simulink model "levitat_model"  (R2024b)
settings: Solver=VariableStepAuto  StartTime=0.0  StopTime=Tsim  RelTol=1e-3
values from neighbouring files (symbols this model uses):
  g = 9.81    [gen_simdata_levit.m]    (also in levitat_data.mat)
  ibar = sqrt((m*g*(mean(z1(idx_start:idx_end))-z0).^2-k0)/Km)    [gen_simdata_levit.m]    (also in levitat_data.mat = 0.990880956794)
  K = place(A,B,pcl)    [gen_simdata_levit.m]
  k0 = 0    [gen_simdata_levit.m]    (also in levitat_data.mat; levitat_id_flcmo.m = x(2))
  Km = magnet_params(1)    [gen_simdata_levit.m]    (also in levitat_data.mat = 0.000210393151874)
  Kt = transducer_params(1)    [gen_simdata_levit.m]    (also in levitat_data.mat = 655.477466063)
  m = 24.197e-3    (= 0.024197)    [gen_simdata_levit.m]    (also in levitat_data.mat)
  Ts = 1e-2    (= 0.01)    [gen_simdata_levit.m]    (also in levitat_data.mat; run_ls.m = d.Ts)
  v0 = transducer_params(2)    [gen_simdata_levit.m]    (also in levitat_data.mat = -40.6780019306)
  zini = z_bar + 2*epsilon*rand - epsilon    [gen_simdata_levit.m]
settings Model: Creator=simon  LastModifiedBy=simon
settings DebuggingCC: UnconnectedInputMsg=warning  UnconnectedOutputMsg=warning  UnconnectedLineMsg=warning
settings ModelReferenceCC: EnableRefExpFcnMdlSchedulingChecks=on
settings RTWCC: GPUComputeCapability=3.5  DLArmComputeVersion=19.05

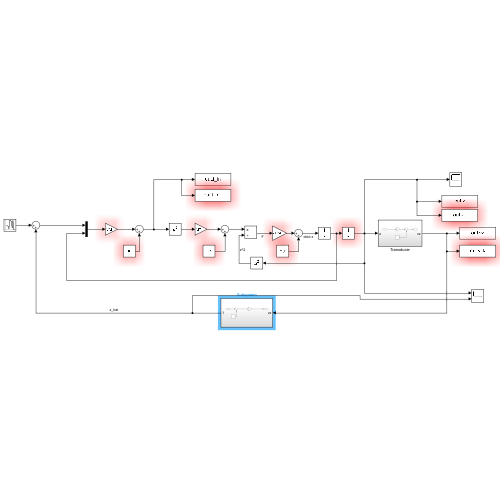
[thumbnail: Simulink's stored preview of the top-level diagram]
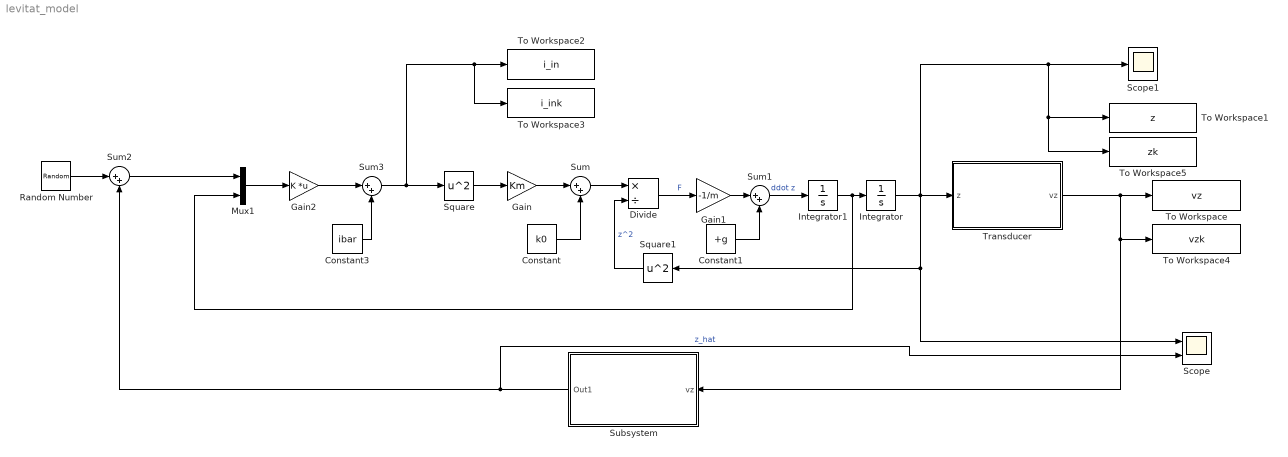
== system levitat_model ==
  Constant : Constant  Value=k0
  Constant1 : Constant  Value=+g
  Constant3 : Constant  Value=ibar
  Divide : Product  Inputs=*/
  Gain : Gain  Gain=Km
  Gain1 : Gain  Gain=-1/m
  Gain2 : Gain  Gain=K  Multiplication=Matrix(K*u)
  Integrator : Integrator  InitialCondition=zini
  Integrator1 : Integrator
  Mux1 : Mux  Inputs=2
  Random Number : RandomNumber  Variance=1e-4  SampleTime=1
  Scope : Scope  NumInputPorts=2
  Scope1 : Scope
  Square : Math  Operator=square
  Square1 : Math  Operator=square
  Subsystem : Subsystem
  Sum{,1..3} (4 alike) : Sum  Inputs=|++
  To Workspace : ToWorkspace  VariableName=vz  SaveFormat=Timeseries  SampleTime=-1
  To Workspace1 : ToWorkspace  VariableName=z  SaveFormat=Timeseries  SampleTime=-1
  To Workspace2 : ToWorkspace  VariableName=i_in  SaveFormat=Timeseries  SampleTime=-1
  To Workspace3 : ToWorkspace  VariableName=i_ink  SaveFormat=Timeseries  SampleTime=Ts
  To Workspace4 : ToWorkspace  VariableName=vzk  SaveFormat=Timeseries  SampleTime=Ts
  To Workspace5 : ToWorkspace  VariableName=zk  SaveFormat=Timeseries  SampleTime=Ts
  Transducer : Subsystem
  wires:
  Square/1 -> Gain/1
  Gain/1 -> Sum/1
  Constant/1 -> Sum/2
  Sum/1 -> Divide/1
  Square1/1 -> Divide/2  "z^2"
  Integrator1/1 -> Mux1/2, Integrator/1
  Sum1/1 -> Integrator1/1  "ddot z"
  Constant1/1 -> Sum1/2
  Gain1/1 -> Sum1/1
  Divide/1 -> Gain1/1  "F"
  Transducer/1(vz) -> To Workspace/1, To Workspace4/1, Subsystem/1(vz)
  Mux1/1 -> Gain2/1
  Sum3/1 -> To Workspace3/1, To Workspace2/1, Square/1
  Gain2/1 -> Sum3/1
  Constant3/1 -> Sum3/2
  Integrator/1 -> Scope/1, Square1/1, To Workspace5/1, To Workspace1/1, Scope1/1, Transducer/1(z)
  Random Number/1 -> Sum2/1
  Sum2/1 -> Mux1/1
  Subsystem/1(Out1) -> Scope/2, Sum2/2  "z_hat"

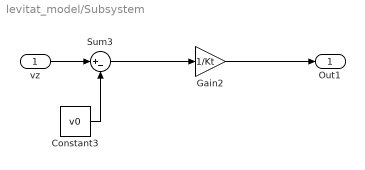
== system levitat_model/Subsystem ==
  vz : Inport
  Constant3 : Constant  Value=v0
  Gain2 : Gain  Gain=1/Kt
  Sum3 : Sum  Inputs=|+-
  Out1 : Outport
  wires:
  Constant3/1 -> Sum3/2
  vz/1 -> Sum3/1
  Sum3/1 -> Gain2/1
  Gain2/1 -> Out1/1

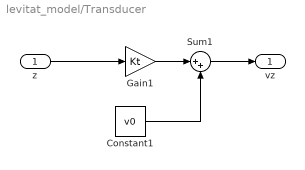
== system levitat_model/Transducer ==
  z : Inport
  Constant1 : Constant  Value=v0
  Gain1 : Gain  Gain=Kt
  Sum1 : Sum  Inputs=|++
  vz : Outport
  wires:
  Gain1/1 -> Sum1/1
  Constant1/1 -> Sum1/2
  z/1 -> Gain1/1
  Sum1/1 -> vz/1
